simulink model "mimo_malha_fechada_descentralizada"  (R2020a)
settings: Solver=VariableStepAuto  StartTime=0.0  StopTime=50000.0  RelTol=1e-3
libraries: cstblocks x6
settings Model: Creator=gabriel  LastModifiedBy=gabriel

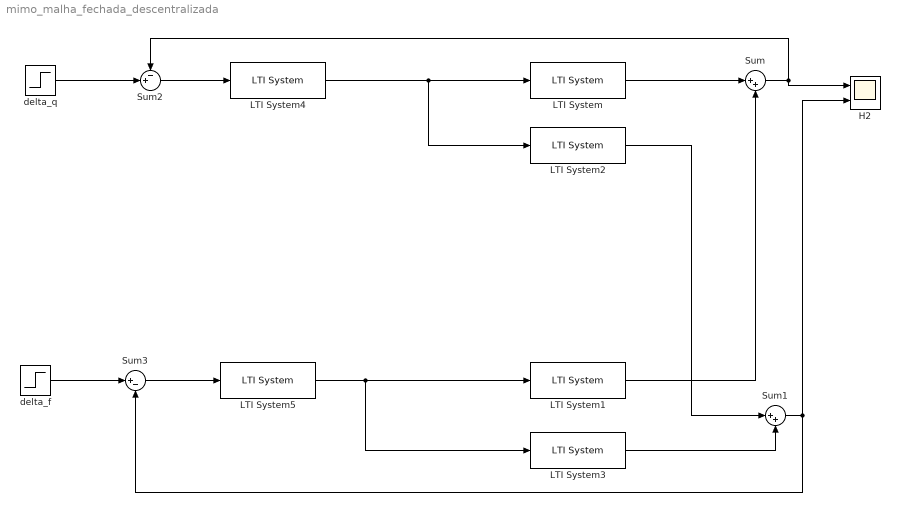
== system mimo_malha_fechada_descentralizada ==
  H2 : Scope  NumInputPorts=2
  LTI System : cstblocks/LTI System  sys=g11  IC=[]
  LTI System1 : cstblocks/LTI System  sys=g12  IC=[]
  LTI System2 : cstblocks/LTI System  sys=g21  IC=[]
  LTI System3 : cstblocks/LTI System  sys=g22  IC=[]
  LTI System4 : cstblocks/LTI System  sys=C1  IC=[]
  LTI System5 : cstblocks/LTI System  sys=C2  IC=[]
  Sum : Sum  Inputs=|++
  Sum1 : Sum  Inputs=|++
  Sum2 : Sum  Inputs=-+|
  Sum3 : Sum  Inputs=|+-
  delta_f : Step  Time=20000  SampleTime=0
  delta_q : Step  SampleTime=0
  wires:
  LTI System2/1 -> Sum1/1
  LTI System3/1 -> Sum1/2
  LTI System1/1 -> Sum/2
  LTI System/1 -> Sum/1
  Sum/1 -> Sum2/1, H2/1
  delta_q/1 -> Sum2/2
  Sum2/1 -> LTI System4/1
  Sum3/1 -> LTI System5/1
  delta_f/1 -> Sum3/1
  Sum1/1 -> Sum3/2, H2/2
  LTI System4/1 -> LTI System2/1, LTI System/1
  LTI System5/1 -> LTI System3/1, LTI System1/1
